simulink model "sampleModel2432"  (R2017a)
settings: Solver=VariableStepAuto  StartTime=0.0  StopTime=10.0  RelTol=1e-3
undefined symbols (not defined in the file or in its folder): DiscIntNeverNeededParam, sigbuilder_block
libraries: simulink x354
(part 3 of 6)

== system sampleModel2432/cfblk229 ==
  cfblk1 : Inport
  cfblk12 : Inport  Port=2
  cfblk13 : Inport  Port=3
  Action Port : ActionPort  ActionType=then
  cfblk10 : UnitDelay  SampleTime=-1
  cfblk11 : simulink/Discrete/Difference  ICPrevInput=0.0  OutMin=[]  OutMax=[]  OutDataTypeStr=Inherit: Inherit via back propagation  OutDataType=fixdt(1, 16)  OutScaling=2^-10  DoSatur=off
  cfblk15 : Delay
  cfblk3 : DiscreteTransferFcn
  cfblk4 : simulink/Discrete/Transfer Fcn Lead or Lag  PoleZ=0.95  ZeroZ=0.75  ICPrevOutput=0.0  ICPrevInput=0.0  DoSatur=off
      settings: SourceProductName=Simulink  SourceProductBaseCode=SL
  cfblk5 : simulink/Discrete/Tapped Delay  vinit=0.0  samptime=-1  NumDelays=1  DelayOrder=Oldest  includeCurrent=off
  cfblk6 : simulink/Continuous/PID Controller (2DOF)  Controller=PID  TimeDomain=Discrete-time  SampleTime=-1  IntegratorMethod=Forward Euler  FilterMethod=Forward Euler  Form=Parallel  UseFilter=on  ControllerParametersSource=internal  P=1  I=1  D=0  N=100  b=1  c=1  InitialConditionSource=internal  InitialConditionForIntegrator=0  InitialConditionForFilter=0  ExternalReset=none  LimitOutput=off  UpperSaturationLimit=inf  LowerSaturationLimit=-inf  LinearizeAsGain=off  AntiWindupMode=none  Kb=1  TrackingMode=off  Kt=1  PParamMin=[]  PParamMax=[]  IParamMin=[]  IParamMax=[]  DParamMin=[]  DParamMax=[]  NParamMin=[]  NParamMax=[]  bParamMin=[]  bParamMax=[]  cParamMin=[]  cParamMax=[]  KbParamMin=[]  KbParamMax=[]  KtParamMin=[]  KtParamMax=[]  POutMin=[]  POutMax=[]  IOutMin=[]  IOutMax=[]  DOutMin=[]  DOutMax=[]  NOutMin=[]  NOutMax=[]  bOutMin=[]  bOutMax=[]  cOutMin=[]  cOutMax=[]  KbOutMin=[]  KbOutMax=[]  KtOutMin=[]  KtOutMax=[]  IntegratorOutMin=[]  IntegratorOutMax=[]  FilterOutMin=[]  FilterOutMax=[]  SumOutMin=[]  SumOutMax=[]  Sum1OutMin=[]  Sum1OutMax=[]  Sum2OutMin=[]  Sum2OutMax=[]  Sum3OutMin=[]  Sum3OutMax=[]  SumI1OutMin=[]  SumI1OutMax=[]  SumI2OutMin=[]  SumI2OutMax=[]  SumI3OutMin=[]  SumI3OutMax=[]  SumDOutMin=[]  SumDOutMax=[]  SaturationOutMin=[]  SaturationOutMax=[]  IntegratorContinuousStateAttributes=''  IntegratorStateMustResolveToSignalObject=off  IntegratorRTWStateStorageClass=Auto  FilterContinuousStateAttributes=''  FilterStateMustResolveToSignalObject=off  FilterRTWStateStorageClass=Auto  DifferentiatorICPrevScaledInput=0  DifferentiatorOutMin=[]  DifferentiatorOutMax=[]  InitialConditionSetting=State (most efficient)
  cfblk7 : simulink/Continuous/PID Controller  Controller=PID  TimeDomain=Discrete-time  SampleTime=-1  IntegratorMethod=Forward Euler  FilterMethod=Forward Euler  Form=Parallel  UseFilter=on  ControllerParametersSource=internal  P=1  I=1  D=0  N=100  InitialConditionSource=internal  InitialConditionForIntegrator=0  InitialConditionForFilter=0  ExternalReset=none  LimitOutput=off  UpperSaturationLimit=inf  LowerSaturationLimit=-inf  LinearizeAsGain=off  AntiWindupMode=none  Kb=1  TrackingMode=off  Kt=1  PParamMin=[]  PParamMax=[]  IParamMin=[]  IParamMax=[]  DParamMin=[]  DParamMax=[]  NParamMin=[]  NParamMax=[]  KbParamMin=[]  KbParamMax=[]  KtParamMin=[]  KtParamMax=[]  POutMin=[]  POutMax=[]  IOutMin=[]  IOutMax=[]  DOutMin=[]  DOutMax=[]  NOutMin=[]  NOutMax=[]  KbOutMin=[]  KbOutMax=[]  KtOutMin=[]  KtOutMax=[]  IntegratorOutMin=[]  IntegratorOutMax=[]  FilterOutMin=[]  FilterOutMax=[]  SumOutMin=[]  SumOutMax=[]  SumI1OutMin=[]  SumI1OutMax=[]  SumI2OutMin=[]  SumI2OutMax=[]  SumI3OutMin=[]  SumI3OutMax=[]  SumDOutMin=[]  SumDOutMax=[]  SaturationOutMin=[]  SaturationOutMax=[]  IntegratorContinuousStateAttributes=''  IntegratorStateMustResolveToSignalObject=off  IntegratorRTWStateStorageClass=Auto  FilterContinuousStateAttributes=''  FilterStateMustResolveToSignalObject=off  FilterRTWStateStorageClass=Auto  DifferentiatorICPrevScaledInput=0  DifferentiatorOutMin=[]  DifferentiatorOutMax=[]  InitialConditionSetting=State (most efficient)
  cfblk8 : simulink/Continuous/PID Controller  Controller=PID  TimeDomain=Discrete-time  SampleTime=-1  IntegratorMethod=Forward Euler  FilterMethod=Forward Euler  Form=Parallel  UseFilter=on  ControllerParametersSource=internal  P=1  I=1  D=0  N=100  InitialConditionSource=internal  InitialConditionForIntegrator=0  InitialConditionForFilter=0  ExternalReset=none  LimitOutput=off  UpperSaturationLimit=inf  LowerSaturationLimit=-inf  LinearizeAsGain=off  AntiWindupMode=none  Kb=1  TrackingMode=off  Kt=1  PParamMin=[]  PParamMax=[]  IParamMin=[]  IParamMax=[]  DParamMin=[]  DParamMax=[]  NParamMin=[]  NParamMax=[]  KbParamMin=[]  KbParamMax=[]  KtParamMin=[]  KtParamMax=[]  POutMin=[]  POutMax=[]  IOutMin=[]  IOutMax=[]  DOutMin=[]  DOutMax=[]  NOutMin=[]  NOutMax=[]  KbOutMin=[]  KbOutMax=[]  KtOutMin=[]  KtOutMax=[]  IntegratorOutMin=[]  IntegratorOutMax=[]  FilterOutMin=[]  FilterOutMax=[]  SumOutMin=[]  SumOutMax=[]  SumI1OutMin=[]  SumI1OutMax=[]  SumI2OutMin=[]  SumI2OutMax=[]  SumI3OutMin=[]  SumI3OutMax=[]  SumDOutMin=[]  SumDOutMax=[]  SaturationOutMin=[]  SaturationOutMax=[]  IntegratorContinuousStateAttributes=''  IntegratorStateMustResolveToSignalObject=off  IntegratorRTWStateStorageClass=Auto  FilterContinuousStateAttributes=''  FilterStateMustResolveToSignalObject=off  FilterRTWStateStorageClass=Auto  DifferentiatorICPrevScaledInput=0  DifferentiatorOutMin=[]  DifferentiatorOutMax=[]  InitialConditionSetting=State (most efficient)
  cfblk9 : DiscreteZeroPole  Poles=[0 0.5]  Gain=1  SampleTime=-1
  cfblk2 : Outport
  cfblk14 : Outport  Port=2
  wires:
  cfblk7/1 -> cfblk8/1
  cfblk5/1 -> cfblk10/1
  cfblk11/1 -> cfblk7/1
  cfblk4/1 -> cfblk9/1
  cfblk8/1 -> cfblk14/1
  cfblk13/1 -> cfblk6/1
  cfblk9/1 -> cfblk5/1
  cfblk1/1 -> cfblk6/2
  cfblk6/1 -> cfblk2/1
  cfblk12/1 -> cfblk3/1
  cfblk3/1 -> cfblk11/1
  cfblk10/1 -> cfblk15/1
  cfblk15/1 -> cfblk4/1

== system sampleModel2432/cfblk230 ==
  cfblk1 : Inport
  Action Port : ActionPort  ActionType=else
  cfblk10 : Subsystem  TreatAsAtomicUnit=on
  cfblk11 : Subsystem  TreatAsAtomicUnit=on
  cfblk12 : Delay
  cfblk3 : DiscreteZeroPole  Poles=[0 0.5]  Gain=1  SampleTime=-1
  cfblk4 : Delay  DelayLengthSource=Input port
      settings: InputPortMap=u0,p1
  cfblk5 : DiscreteZeroPole  Poles=[0 0.5]  Gain=1  SampleTime=-1
  cfblk6 : simulink/Discrete/Transfer Fcn Lead or Lag  PoleZ=0.95  ZeroZ=0.75  ICPrevOutput=0.0  ICPrevInput=0.0  DoSatur=off
      settings: SourceProductName=Simulink  SourceProductBaseCode=SL
  cfblk7 : DiscreteIntegrator  InitialConditionSetting=State (most efficient)  SampleTime=-1  ICPrevOutput=DiscIntNeverNeededParam  ICPrevScaledInput=DiscIntNeverNeededParam
  cfblk8 : simulink/Continuous/PID Controller  Controller=PID  TimeDomain=Discrete-time  SampleTime=-1  IntegratorMethod=Forward Euler  FilterMethod=Forward Euler  Form=Parallel  UseFilter=on  ControllerParametersSource=internal  P=1  I=1  D=0  N=100  InitialConditionSource=internal  InitialConditionForIntegrator=0  InitialConditionForFilter=0  ExternalReset=none  LimitOutput=off  UpperSaturationLimit=inf  LowerSaturationLimit=-inf  LinearizeAsGain=off  AntiWindupMode=none  Kb=1  TrackingMode=off  Kt=1  PParamMin=[]  PParamMax=[]  IParamMin=[]  IParamMax=[]  DParamMin=[]  DParamMax=[]  NParamMin=[]  NParamMax=[]  KbParamMin=[]  KbParamMax=[]  KtParamMin=[]  KtParamMax=[]  POutMin=[]  POutMax=[]  IOutMin=[]  IOutMax=[]  DOutMin=[]  DOutMax=[]  NOutMin=[]  NOutMax=[]  KbOutMin=[]  KbOutMax=[]  KtOutMin=[]  KtOutMax=[]  IntegratorOutMin=[]  IntegratorOutMax=[]  FilterOutMin=[]  FilterOutMax=[]  SumOutMin=[]  SumOutMax=[]  SumI1OutMin=[]  SumI1OutMax=[]  SumI2OutMin=[]  SumI2OutMax=[]  SumI3OutMin=[]  SumI3OutMax=[]  SumDOutMin=[]  SumDOutMax=[]  SaturationOutMin=[]  SaturationOutMax=[]  IntegratorContinuousStateAttributes=''  IntegratorStateMustResolveToSignalObject=off  IntegratorRTWStateStorageClass=Auto  FilterContinuousStateAttributes=''  FilterStateMustResolveToSignalObject=off  FilterRTWStateStorageClass=Auto  DifferentiatorICPrevScaledInput=0  DifferentiatorOutMin=[]  DifferentiatorOutMax=[]  InitialConditionSetting=State (most efficient)
  cfblk9 : If  SampleTime=1
  cfblk2 : Outport
  wires:
  cfblk7/1 -> cfblk3/1
  cfblk10/1(cfblk2) -> cfblk7/1
  cfblk10/2(cfblk11) -> cfblk11/1(cfblk1)
  cfblk8/1 -> cfblk6/1
  cfblk5/1 -> cfblk2/1
  cfblk1/1 -> cfblk9/1
  cfblk3/1 -> cfblk5/1
  cfblk10/3(cfblk12) -> cfblk4/1
  cfblk11/1(cfblk2) -> cfblk8/1
  cfblk11/2(cfblk10) -> cfblk4/2
  cfblk9/1 -> cfblk10/Action
  cfblk9/2 -> cfblk11/Action
  cfblk6/1 -> cfblk12/1
  cfblk12/1 -> cfblk10/1(cfblk1)

== system sampleModel2432/cfblk231 ==
  cfblk1 : Inport
  cfblk11 : Inport  Port=2
  cfblk12 : Inport  Port=3
  Action Port : ActionPort  ActionType=then
  cfblk10 : If  SampleTime=1
  cfblk14 : Subsystem  TreatAsAtomicUnit=on
  cfblk15 : Subsystem  TreatAsAtomicUnit=on
  cfblk16 : Delay
  cfblk17 : Delay
  cfblk3 : Delay
  cfblk4 : simulink/Discrete/Transfer Fcn First Order  PoleZ=0.95  ICPrevOutput=0.0  DoSatur=off
      settings: SourceProductName=Simulink
  cfblk5 : simulink/Discrete/Difference  ICPrevInput=0.0  OutMin=[]  OutMax=[]  OutDataTypeStr=Inherit: Inherit via back propagation  OutDataType=fixdt(1, 16)  OutScaling=2^-10  DoSatur=off
  cfblk6 : DiscreteIntegrator  InitialConditionSetting=State (most efficient)  SampleTime=-1  ICPrevOutput=DiscIntNeverNeededParam  ICPrevScaledInput=DiscIntNeverNeededParam
  cfblk7 : DiscreteFilter
  cfblk8 : DiscreteFir
  cfblk9 : simulink/Discrete/Tapped Delay  vinit=0.0  samptime=-1  NumDelays=1  DelayOrder=Oldest  includeCurrent=off
  cfblk2 : Outport
  cfblk13 : Outport  Port=2
  wires:
  cfblk11/1 -> cfblk6/1
  cfblk5/1 -> cfblk3/1
  cfblk4/1 -> cfblk5/1
  cfblk14/1(cfblk2) -> cfblk4/1
  cfblk9/1 -> cfblk13/1
  cfblk6/1 -> cfblk14/2(cfblk6)
  cfblk1/1 -> cfblk15/1(cfblk1)
  cfblk12/1 -> cfblk14/3(cfblk7)
  cfblk15/1(cfblk2) -> cfblk8/1
  cfblk14/2(cfblk10) -> cfblk9/1
  cfblk15/2(cfblk6) -> cfblk7/1
  cfblk14/3(cfblk11) -> cfblk2/1
  cfblk15/3(cfblk7) -> cfblk14/4(cfblk8)
  cfblk15/4(cfblk8) -> cfblk14/5(cfblk9)
  cfblk10/1 -> cfblk14/Action
  cfblk10/2 -> cfblk15/Action
  cfblk3/1 -> cfblk16/1
  cfblk16/1 -> cfblk14/1(cfblk1)
  cfblk8/1 -> cfblk17/1
  cfblk17/1 -> cfblk10/1

== system sampleModel2432/cfblk232 ==
  cfblk1 : Inport
  cfblk7 : Inport  Port=2
  Action Port : ActionPort  ActionType=else
  cfblk3 : simulink/Continuous/PID Controller (2DOF)  Controller=PID  TimeDomain=Discrete-time  SampleTime=-1  IntegratorMethod=Forward Euler  FilterMethod=Forward Euler  Form=Parallel  UseFilter=on  ControllerParametersSource=internal  P=1  I=1  D=0  N=100  b=1  c=1  InitialConditionSource=internal  InitialConditionForIntegrator=0  InitialConditionForFilter=0  ExternalReset=none  LimitOutput=off  UpperSaturationLimit=inf  LowerSaturationLimit=-inf  LinearizeAsGain=off  AntiWindupMode=none  Kb=1  TrackingMode=off  Kt=1  PParamMin=[]  PParamMax=[]  IParamMin=[]  IParamMax=[]  DParamMin=[]  DParamMax=[]  NParamMin=[]  NParamMax=[]  bParamMin=[]  bParamMax=[]  cParamMin=[]  cParamMax=[]  KbParamMin=[]  KbParamMax=[]  KtParamMin=[]  KtParamMax=[]  POutMin=[]  POutMax=[]  IOutMin=[]  IOutMax=[]  DOutMin=[]  DOutMax=[]  NOutMin=[]  NOutMax=[]  bOutMin=[]  bOutMax=[]  cOutMin=[]  cOutMax=[]  KbOutMin=[]  KbOutMax=[]  KtOutMin=[]  KtOutMax=[]  IntegratorOutMin=[]  IntegratorOutMax=[]  FilterOutMin=[]  FilterOutMax=[]  SumOutMin=[]  SumOutMax=[]  Sum1OutMin=[]  Sum1OutMax=[]  Sum2OutMin=[]  Sum2OutMax=[]  Sum3OutMin=[]  Sum3OutMax=[]  SumI1OutMin=[]  SumI1OutMax=[]  SumI2OutMin=[]  SumI2OutMax=[]  SumI3OutMin=[]  SumI3OutMax=[]  SumDOutMin=[]  SumDOutMax=[]  SaturationOutMin=[]  SaturationOutMax=[]  IntegratorContinuousStateAttributes=''  IntegratorStateMustResolveToSignalObject=off  IntegratorRTWStateStorageClass=Auto  FilterContinuousStateAttributes=''  FilterStateMustResolveToSignalObject=off  FilterRTWStateStorageClass=Auto  DifferentiatorICPrevScaledInput=0  DifferentiatorOutMin=[]  DifferentiatorOutMax=[]  InitialConditionSetting=State (most efficient)
  cfblk4 : simulink/Discrete/Transfer Fcn First Order  PoleZ=0.95  ICPrevOutput=0.0  DoSatur=off
      settings: SourceProductName=Simulink
  cfblk5 : Delay
  cfblk6 : simulink/Discrete/Difference  ICPrevInput=0.0  OutMin=[]  OutMax=[]  OutDataTypeStr=Inherit: Inherit via back propagation  OutDataType=fixdt(1, 16)  OutScaling=2^-10  DoSatur=off
  cfblk8 : Delay
  cfblk2 : Outport
  wires:
  cfblk4/1 -> cfblk6/1
  cfblk7/1 -> cfblk3/1
  cfblk3/1 -> cfblk2/1
  cfblk1/1 -> cfblk5/1
  cfblk5/1 -> cfblk3/2
  cfblk6/1 -> cfblk8/1
  cfblk8/1 -> cfblk4/1

== system sampleModel2432/cfblk233 ==
  cfblk1 : Inport
  Action Port : ActionPort  ActionType=then
  cfblk10 : DiscreteIntegrator  InitialConditionSetting=State (most efficient)  SampleTime=-1  ICPrevOutput=DiscIntNeverNeededParam  ICPrevScaledInput=DiscIntNeverNeededParam
  cfblk{5,8..9,11..12} (5 alike) : DiscreteFir
  cfblk13 : simulink/Continuous/PID Controller  Controller=PID  TimeDomain=Discrete-time  SampleTime=-1  IntegratorMethod=Forward Euler  FilterMethod=Forward Euler  Form=Parallel  UseFilter=on  ControllerParametersSource=internal  P=1  I=1  D=0  N=100  InitialConditionSource=internal  InitialConditionForIntegrator=0  InitialConditionForFilter=0  ExternalReset=none  LimitOutput=off  UpperSaturationLimit=inf  LowerSaturationLimit=-inf  LinearizeAsGain=off  AntiWindupMode=none  Kb=1  TrackingMode=off  Kt=1  PParamMin=[]  PParamMax=[]  IParamMin=[]  IParamMax=[]  DParamMin=[]  DParamMax=[]  NParamMin=[]  NParamMax=[]  KbParamMin=[]  KbParamMax=[]  KtParamMin=[]  KtParamMax=[]  POutMin=[]  POutMax=[]  IOutMin=[]  IOutMax=[]  DOutMin=[]  DOutMax=[]  NOutMin=[]  NOutMax=[]  KbOutMin=[]  KbOutMax=[]  KtOutMin=[]  KtOutMax=[]  IntegratorOutMin=[]  IntegratorOutMax=[]  FilterOutMin=[]  FilterOutMax=[]  SumOutMin=[]  SumOutMax=[]  SumI1OutMin=[]  SumI1OutMax=[]  SumI2OutMin=[]  SumI2OutMax=[]  SumI3OutMin=[]  SumI3OutMax=[]  SumDOutMin=[]  SumDOutMax=[]  SaturationOutMin=[]  SaturationOutMax=[]  IntegratorContinuousStateAttributes=''  IntegratorStateMustResolveToSignalObject=off  IntegratorRTWStateStorageClass=Auto  FilterContinuousStateAttributes=''  FilterStateMustResolveToSignalObject=off  FilterRTWStateStorageClass=Auto  DifferentiatorICPrevScaledInput=0  DifferentiatorOutMin=[]  DifferentiatorOutMax=[]  InitialConditionSetting=State (most efficient)
  cfblk14 : DiscreteZeroPole  Poles=[0 0.5]  Gain=1  SampleTime=-1
  cfblk15 : Delay
  cfblk16 : Delay
  cfblk3 : simulink/Discrete/Tapped Delay  vinit=0.0  samptime=-1  NumDelays=1  DelayOrder=Oldest  includeCurrent=off
  cfblk4 : simulink/Discrete/Transfer Fcn First Order  PoleZ=0.95  ICPrevOutput=0.0  DoSatur=off
      settings: SourceProductName=Simulink
  cfblk6 : simulink/Discrete/Transfer Fcn Lead or Lag  PoleZ=0.95  ZeroZ=0.75  ICPrevOutput=0.0  ICPrevInput=0.0  DoSatur=off
      settings: SourceProductName=Simulink  SourceProductBaseCode=SL
  cfblk7 : simulink/Discrete/Transfer Fcn Lead or Lag  PoleZ=0.95  ZeroZ=0.75  ICPrevOutput=0.0  ICPrevInput=0.0  DoSatur=off
      settings: SourceProductName=Simulink  SourceProductBaseCode=SL
  cfblk2 : Outport
  wires:
  cfblk14/1 -> cfblk9/1
  cfblk3/1 -> cfblk12/1
  cfblk7/1 -> cfblk6/1
  cfblk9/1 -> cfblk10/1
  cfblk12/1 -> cfblk2/1
  cfblk8/1 -> cfblk11/1
  cfblk6/1 -> cfblk13/1
  cfblk4/1 -> cfblk14/1
  cfblk5/1 -> cfblk8/1
  cfblk1/1 -> cfblk3/1
  cfblk10/1 -> cfblk7/1
  cfblk13/1 -> cfblk15/1
  cfblk15/1 -> cfblk4/1
  cfblk11/1 -> cfblk16/1
  cfblk16/1 -> cfblk5/1

== system sampleModel2432/cfblk234 ==
  cfblk1 : Inport
  cfblk7 : Inport  Port=2
  Action Port : ActionPort  ActionType=else
  cfblk10 : Delay
  cfblk11 : Delay
  cfblk3 : simulink/Discrete/Difference  ICPrevInput=0.0  OutMin=[]  OutMax=[]  OutDataTypeStr=Inherit: Inherit via back propagation  OutDataType=fixdt(1, 16)  OutScaling=2^-10  DoSatur=off
  cfblk4 : simulink/Discrete/Difference  ICPrevInput=0.0  OutMin=[]  OutMax=[]  OutDataTypeStr=Inherit: Inherit via back propagation  OutDataType=fixdt(1, 16)  OutScaling=2^-10  DoSatur=off
  cfblk5 : Delay
  cfblk6 : If  SampleTime=1
  cfblk8 : Subsystem  TreatAsAtomicUnit=on
  cfblk9 : Subsystem  TreatAsAtomicUnit=on
  cfblk2 : Outport
  wires:
  cfblk8/1(cfblk2) -> cfblk5/1
  cfblk7/1 -> cfblk8/1(cfblk1)
  cfblk4/1 -> cfblk2/1
  cfblk1/1 -> cfblk4/1
  cfblk3/1 -> cfblk9/1(cfblk1)
  cfblk6/1 -> cfblk8/Action
  cfblk6/2 -> cfblk9/Action
  cfblk5/1 -> cfblk10/1
  cfblk10/1 -> cfblk3/1
  cfblk9/1(cfblk2) -> cfblk11/1
  cfblk11/1 -> cfblk6/1

== system sampleModel2432/cfblk235 ==
  cfblk1 : Inport
  Action Port : ActionPort  ActionType=then
  cfblk10 : Delay
  cfblk3 : Delay  ShowEnablePort=on
      settings: InputPortMap=u0,e6
  cfblk4 : DiscreteIntegrator  InitialConditionSetting=State (most efficient)  SampleTime=-1  ICPrevOutput=DiscIntNeverNeededParam  ICPrevScaledInput=DiscIntNeverNeededParam
  cfblk5 : simulink/Continuous/PID Controller  Controller=PID  TimeDomain=Discrete-time  SampleTime=-1  IntegratorMethod=Forward Euler  FilterMethod=Forward Euler  Form=Parallel  UseFilter=on  ControllerParametersSource=internal  P=1  I=1  D=0  N=100  InitialConditionSource=internal  InitialConditionForIntegrator=0  InitialConditionForFilter=0  ExternalReset=none  LimitOutput=off  UpperSaturationLimit=inf  LowerSaturationLimit=-inf  LinearizeAsGain=off  AntiWindupMode=none  Kb=1  TrackingMode=off  Kt=1  PParamMin=[]  PParamMax=[]  IParamMin=[]  IParamMax=[]  DParamMin=[]  DParamMax=[]  NParamMin=[]  NParamMax=[]  KbParamMin=[]  KbParamMax=[]  KtParamMin=[]  KtParamMax=[]  POutMin=[]  POutMax=[]  IOutMin=[]  IOutMax=[]  DOutMin=[]  DOutMax=[]  NOutMin=[]  NOutMax=[]  KbOutMin=[]  KbOutMax=[]  KtOutMin=[]  KtOutMax=[]  IntegratorOutMin=[]  IntegratorOutMax=[]  FilterOutMin=[]  FilterOutMax=[]  SumOutMin=[]  SumOutMax=[]  SumI1OutMin=[]  SumI1OutMax=[]  SumI2OutMin=[]  SumI2OutMax=[]  SumI3OutMin=[]  SumI3OutMax=[]  SumDOutMin=[]  SumDOutMax=[]  SaturationOutMin=[]  SaturationOutMax=[]  IntegratorContinuousStateAttributes=''  IntegratorStateMustResolveToSignalObject=off  IntegratorRTWStateStorageClass=Auto  FilterContinuousStateAttributes=''  FilterStateMustResolveToSignalObject=off  FilterRTWStateStorageClass=Auto  DifferentiatorICPrevScaledInput=0  DifferentiatorOutMin=[]  DifferentiatorOutMax=[]  InitialConditionSetting=State (most efficient)
  cfblk6 : Delay  ShowEnablePort=on
      settings: InputPortMap=u0,e6
  cfblk7 : Delay
  cfblk9 : Delay
  cfblk2 : Outport
  cfblk8 : Outport  Port=2
  wires:
  cfblk1/1 -> cfblk6/1, cfblk2/1
  cfblk7/1 -> cfblk8/1, cfblk6/2, cfblk10/1
  cfblk3/1 -> cfblk5/1
  cfblk4/1 -> cfblk7/1
  cfblk6/1 -> cfblk3/2
  cfblk5/1 -> cfblk9/1
  cfblk9/1 -> cfblk3/1
  cfblk10/1 -> cfblk4/1

== system sampleModel2432/cfblk236 ==
  cfblk1 : Inport
  Action Port : ActionPort  ActionType=else
  cfblk{9..12} (4 alike) : DiscreteIntegrator  InitialConditionSetting=State (most efficient)  SampleTime=-1  ICPrevOutput=DiscIntNeverNeededParam  ICPrevScaledInput=DiscIntNeverNeededParam
  cfblk13 : simulink/Discrete/Transfer Fcn First Order  PoleZ=0.95  ICPrevOutput=0.0  DoSatur=off
      settings: SourceProductName=Simulink
  cfblk3 : simulink/Continuous/PID Controller  Controller=PID  TimeDomain=Discrete-time  SampleTime=-1  IntegratorMethod=Forward Euler  FilterMethod=Forward Euler  Form=Parallel  UseFilter=on  ControllerParametersSource=internal  P=1  I=1  D=0  N=100  InitialConditionSource=internal  InitialConditionForIntegrator=0  InitialConditionForFilter=0  ExternalReset=none  LimitOutput=off  UpperSaturationLimit=inf  LowerSaturationLimit=-inf  LinearizeAsGain=off  AntiWindupMode=none  Kb=1  TrackingMode=off  Kt=1  PParamMin=[]  PParamMax=[]  IParamMin=[]  IParamMax=[]  DParamMin=[]  DParamMax=[]  NParamMin=[]  NParamMax=[]  KbParamMin=[]  KbParamMax=[]  KtParamMin=[]  KtParamMax=[]  POutMin=[]  POutMax=[]  IOutMin=[]  IOutMax=[]  DOutMin=[]  DOutMax=[]  NOutMin=[]  NOutMax=[]  KbOutMin=[]  KbOutMax=[]  KtOutMin=[]  KtOutMax=[]  IntegratorOutMin=[]  IntegratorOutMax=[]  FilterOutMin=[]  FilterOutMax=[]  SumOutMin=[]  SumOutMax=[]  SumI1OutMin=[]  SumI1OutMax=[]  SumI2OutMin=[]  SumI2OutMax=[]  SumI3OutMin=[]  SumI3OutMax=[]  SumDOutMin=[]  SumDOutMax=[]  SaturationOutMin=[]  SaturationOutMax=[]  IntegratorContinuousStateAttributes=''  IntegratorStateMustResolveToSignalObject=off  IntegratorRTWStateStorageClass=Auto  FilterContinuousStateAttributes=''  FilterStateMustResolveToSignalObject=off  FilterRTWStateStorageClass=Auto  DifferentiatorICPrevScaledInput=0  DifferentiatorOutMin=[]  DifferentiatorOutMax=[]  InitialConditionSetting=State (most efficient)
  cfblk4 : simulink/Discrete/Tapped Delay  vinit=0.0  samptime=-1  NumDelays=1  DelayOrder=Oldest  includeCurrent=off
  cfblk5 : Delay  DelayLengthSource=Input port
      settings: InputPortMap=u0,p1
  cfblk6 : Delay  ShowEnablePort=on
      settings: InputPortMap=u0,e6
  cfblk7 : Delay
  cfblk8 : DiscreteTransferFcn
  cfblk2 : Outport
  wires:
  cfblk3/1 -> cfblk4/1, cfblk13/1
  cfblk1/1 -> cfblk3/1, cfblk6/2
  cfblk9/1 -> cfblk8/1
  cfblk8/1 -> cfblk10/1
  cfblk5/1 -> cfblk2/1
  cfblk12/1 -> cfblk11/1
  cfblk10/1 -> cfblk12/1
  cfblk7/1 -> cfblk5/1
  cfblk6/1 -> cfblk7/1
  cfblk13/1 -> cfblk9/1
  cfblk4/1 -> cfblk6/1
  cfblk11/1 -> cfblk5/2

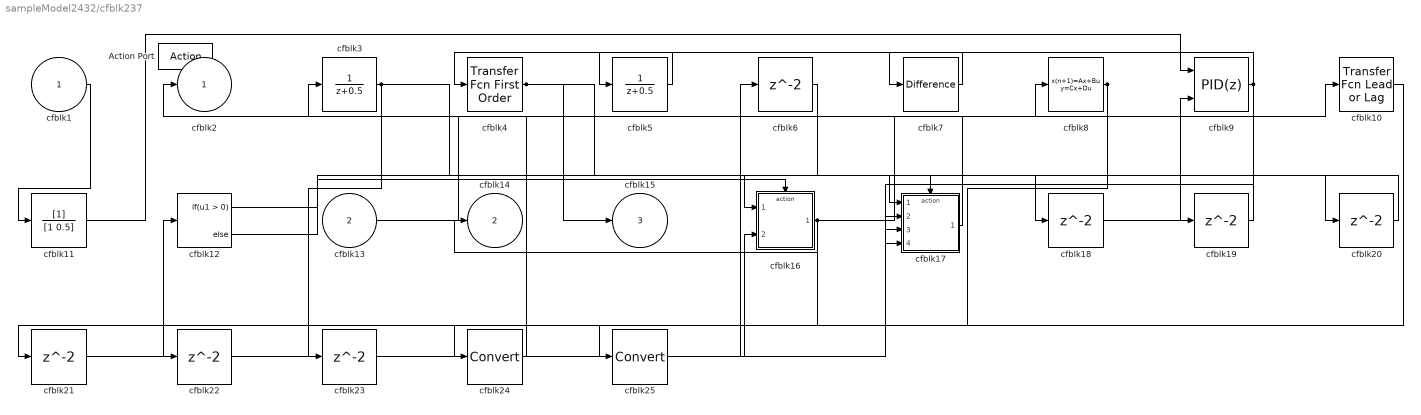
== system sampleModel2432/cfblk237 ==
  cfblk1 : Inport
  cfblk13 : Inport  Port=2
  Action Port : ActionPort  ActionType=then
  cfblk10 : simulink/Discrete/Transfer Fcn Lead or Lag  PoleZ=0.95  ZeroZ=0.75  ICPrevOutput=0.0  ICPrevInput=0.0  DoSatur=off
      settings: SourceProductName=Simulink  SourceProductBaseCode=SL
  cfblk11 : DiscreteFilter
  cfblk12 : If  SampleTime=1
  cfblk16 : Subsystem  TreatAsAtomicUnit=on
  cfblk17 : Subsystem  TreatAsAtomicUnit=on
  cfblk{6,18..23} (7 alike) : Delay
  cfblk24 : DataTypeConversion
  cfblk25 : DataTypeConversion
  cfblk3 : DiscreteTransferFcn
  cfblk4 : simulink/Discrete/Transfer Fcn First Order  PoleZ=0.95  ICPrevOutput=0.0  DoSatur=off
      settings: SourceProductName=Simulink
  cfblk5 : DiscreteTransferFcn
  cfblk7 : simulink/Discrete/Difference  ICPrevInput=0.0  OutMin=[]  OutMax=[]  OutDataTypeStr=Inherit: Inherit via back propagation  OutDataType=fixdt(1, 16)  OutScaling=2^-10  DoSatur=off
  cfblk8 : DiscreteStateSpace  SampleTime=-1
  cfblk9 : simulink/Continuous/PID Controller (2DOF)  Controller=PID  TimeDomain=Discrete-time  SampleTime=-1  IntegratorMethod=Forward Euler  FilterMethod=Forward Euler  Form=Parallel  UseFilter=on  ControllerParametersSource=internal  P=1  I=1  D=0  N=100  b=1  c=1  InitialConditionSource=internal  InitialConditionForIntegrator=0  InitialConditionForFilter=0  ExternalReset=none  LimitOutput=off  UpperSaturationLimit=inf  LowerSaturationLimit=-inf  LinearizeAsGain=off  AntiWindupMode=none  Kb=1  TrackingMode=off  Kt=1  PParamMin=[]  PParamMax=[]  IParamMin=[]  IParamMax=[]  DParamMin=[]  DParamMax=[]  NParamMin=[]  NParamMax=[]  bParamMin=[]  bParamMax=[]  cParamMin=[]  cParamMax=[]  KbParamMin=[]  KbParamMax=[]  KtParamMin=[]  KtParamMax=[]  POutMin=[]  POutMax=[]  IOutMin=[]  IOutMax=[]  DOutMin=[]  DOutMax=[]  NOutMin=[]  NOutMax=[]  bOutMin=[]  bOutMax=[]  cOutMin=[]  cOutMax=[]  KbOutMin=[]  KbOutMax=[]  KtOutMin=[]  KtOutMax=[]  IntegratorOutMin=[]  IntegratorOutMax=[]  FilterOutMin=[]  FilterOutMax=[]  SumOutMin=[]  SumOutMax=[]  Sum1OutMin=[]  Sum1OutMax=[]  Sum2OutMin=[]  Sum2OutMax=[]  Sum3OutMin=[]  Sum3OutMax=[]  SumI1OutMin=[]  SumI1OutMax=[]  SumI2OutMin=[]  SumI2OutMax=[]  SumI3OutMin=[]  SumI3OutMax=[]  SumDOutMin=[]  SumDOutMax=[]  SaturationOutMin=[]  SaturationOutMax=[]  IntegratorContinuousStateAttributes=''  IntegratorStateMustResolveToSignalObject=off  IntegratorRTWStateStorageClass=Auto  FilterContinuousStateAttributes=''  FilterStateMustResolveToSignalObject=off  FilterRTWStateStorageClass=Auto  DifferentiatorICPrevScaledInput=0  DifferentiatorOutMin=[]  DifferentiatorOutMax=[]  InitialConditionSetting=State (most efficient)
  cfblk2 : Outport
  cfblk14 : Outport  Port=2
  cfblk15 : Outport  Port=3
  wires:
  cfblk4/1 -> cfblk15/1, cfblk18/1
  cfblk1/1 -> cfblk11/1
  cfblk5/1 -> cfblk4/1
  cfblk16/1(cfblk2) -> cfblk10/1, cfblk14/1, cfblk22/1
  cfblk8/1 -> cfblk17/2(cfblk10), cfblk25/1
  cfblk7/1 -> cfblk5/1
  cfblk13/1 -> cfblk8/1
  cfblk11/1 -> cfblk9/1
  cfblk17/1(cfblk2) -> cfblk3/1
  cfblk9/1 -> cfblk7/1, cfblk17/4(cfblk12)
  cfblk3/1 -> cfblk19/1, cfblk20/1, cfblk23/1
  cfblk12/1 -> cfblk16/Action
  cfblk12/2 -> cfblk17/Action
  cfblk18/1 -> cfblk9/2
  cfblk19/1 -> cfblk17/1(cfblk1)
  cfblk20/1 -> cfblk16/1(cfblk1)
  cfblk10/1 -> cfblk21/1
  cfblk21/1 -> cfblk12/1
  cfblk22/1 -> cfblk17/3(cfblk11)
  cfblk23/1 -> cfblk16/2(cfblk16)
  cfblk6/1 -> cfblk24/1
  cfblk24/1 -> cfblk2/1
  cfblk25/1 -> cfblk6/1

== system sampleModel2432/cfblk238 ==
  cfblk1 : Inport
  cfblk12 : Inport  Port=2
  Action Port : ActionPort  ActionType=else
  cfblk10 : DiscreteIntegrator  InitialConditionSetting=State (most efficient)  SampleTime=-1  ICPrevOutput=DiscIntNeverNeededParam  ICPrevScaledInput=DiscIntNeverNeededParam
  cfblk11 : Delay  ShowEnablePort=on
      settings: InputPortMap=u0,e6
  cfblk16 : Delay
  cfblk17 : Delay
  cfblk3 : DiscreteFilter
  cfblk4 : simulink/Discrete/Difference  ICPrevInput=0.0  OutMin=[]  OutMax=[]  OutDataTypeStr=Inherit: Inherit via back propagation  OutDataType=fixdt(1, 16)  OutScaling=2^-10  DoSatur=off
  cfblk5 : simulink/Continuous/PID Controller  Controller=PID  TimeDomain=Discrete-time  SampleTime=-1  IntegratorMethod=Forward Euler  FilterMethod=Forward Euler  Form=Parallel  UseFilter=on  ControllerParametersSource=internal  P=1  I=1  D=0  N=100  InitialConditionSource=internal  InitialConditionForIntegrator=0  InitialConditionForFilter=0  ExternalReset=none  LimitOutput=off  UpperSaturationLimit=inf  LowerSaturationLimit=-inf  LinearizeAsGain=off  AntiWindupMode=none  Kb=1  TrackingMode=off  Kt=1  PParamMin=[]  PParamMax=[]  IParamMin=[]  IParamMax=[]  DParamMin=[]  DParamMax=[]  NParamMin=[]  NParamMax=[]  KbParamMin=[]  KbParamMax=[]  KtParamMin=[]  KtParamMax=[]  POutMin=[]  POutMax=[]  IOutMin=[]  IOutMax=[]  DOutMin=[]  DOutMax=[]  NOutMin=[]  NOutMax=[]  KbOutMin=[]  KbOutMax=[]  KtOutMin=[]  KtOutMax=[]  IntegratorOutMin=[]  IntegratorOutMax=[]  FilterOutMin=[]  FilterOutMax=[]  SumOutMin=[]  SumOutMax=[]  SumI1OutMin=[]  SumI1OutMax=[]  SumI2OutMin=[]  SumI2OutMax=[]  SumI3OutMin=[]  SumI3OutMax=[]  SumDOutMin=[]  SumDOutMax=[]  SaturationOutMin=[]  SaturationOutMax=[]  IntegratorContinuousStateAttributes=''  IntegratorStateMustResolveToSignalObject=off  IntegratorRTWStateStorageClass=Auto  FilterContinuousStateAttributes=''  FilterStateMustResolveToSignalObject=off  FilterRTWStateStorageClass=Auto  DifferentiatorICPrevScaledInput=0  DifferentiatorOutMin=[]  DifferentiatorOutMax=[]  InitialConditionSetting=State (most efficient)
  cfblk6 : simulink/Continuous/PID Controller (2DOF)  Controller=PID  TimeDomain=Discrete-time  SampleTime=-1  IntegratorMethod=Forward Euler  FilterMethod=Forward Euler  Form=Parallel  UseFilter=on  ControllerParametersSource=internal  P=1  I=1  D=0  N=100  b=1  c=1  InitialConditionSource=internal  InitialConditionForIntegrator=0  InitialConditionForFilter=0  ExternalReset=none  LimitOutput=off  UpperSaturationLimit=inf  LowerSaturationLimit=-inf  LinearizeAsGain=off  AntiWindupMode=none  Kb=1  TrackingMode=off  Kt=1  PParamMin=[]  PParamMax=[]  IParamMin=[]  IParamMax=[]  DParamMin=[]  DParamMax=[]  NParamMin=[]  NParamMax=[]  bParamMin=[]  bParamMax=[]  cParamMin=[]  cParamMax=[]  KbParamMin=[]  KbParamMax=[]  KtParamMin=[]  KtParamMax=[]  POutMin=[]  POutMax=[]  IOutMin=[]  IOutMax=[]  DOutMin=[]  DOutMax=[]  NOutMin=[]  NOutMax=[]  bOutMin=[]  bOutMax=[]  cOutMin=[]  cOutMax=[]  KbOutMin=[]  KbOutMax=[]  KtOutMin=[]  KtOutMax=[]  IntegratorOutMin=[]  IntegratorOutMax=[]  FilterOutMin=[]  FilterOutMax=[]  SumOutMin=[]  SumOutMax=[]  Sum1OutMin=[]  Sum1OutMax=[]  Sum2OutMin=[]  Sum2OutMax=[]  Sum3OutMin=[]  Sum3OutMax=[]  SumI1OutMin=[]  SumI1OutMax=[]  SumI2OutMin=[]  SumI2OutMax=[]  SumI3OutMin=[]  SumI3OutMax=[]  SumDOutMin=[]  SumDOutMax=[]  SaturationOutMin=[]  SaturationOutMax=[]  IntegratorContinuousStateAttributes=''  IntegratorStateMustResolveToSignalObject=off  IntegratorRTWStateStorageClass=Auto  FilterContinuousStateAttributes=''  FilterStateMustResolveToSignalObject=off  FilterRTWStateStorageClass=Auto  DifferentiatorICPrevScaledInput=0  DifferentiatorOutMin=[]  DifferentiatorOutMax=[]  InitialConditionSetting=State (most efficient)
  cfblk7 : simulink/Discrete/Transfer Fcn First Order  PoleZ=0.95  ICPrevOutput=0.0  DoSatur=off
      settings: SourceProductName=Simulink
  cfblk8 : simulink/Discrete/Transfer Fcn First Order  PoleZ=0.95  ICPrevOutput=0.0  DoSatur=off
      settings: SourceProductName=Simulink
  cfblk9 : UnitDelay  SampleTime=-1
  cfblk2 : Outport
  cfblk13 : Outport  Port=2
  cfblk14 : Outport  Port=3
  cfblk15 : Outport  Port=4
  wires:
  cfblk5/1 -> cfblk11/1
  cfblk6/1 -> cfblk15/1, cfblk16/1
  cfblk9/1 -> cfblk14/1
  cfblk11/1 -> cfblk7/1, cfblk10/1, cfblk6/2
  cfblk4/1 -> cfblk5/1
  cfblk1/1 -> cfblk8/1
  cfblk3/1 -> cfblk2/1, cfblk4/1
  cfblk12/1 -> cfblk13/1
  cfblk7/1 -> cfblk6/1
  cfblk8/1 -> cfblk9/1
  cfblk16/1 -> cfblk11/2
  cfblk10/1 -> cfblk17/1
  cfblk17/1 -> cfblk3/1

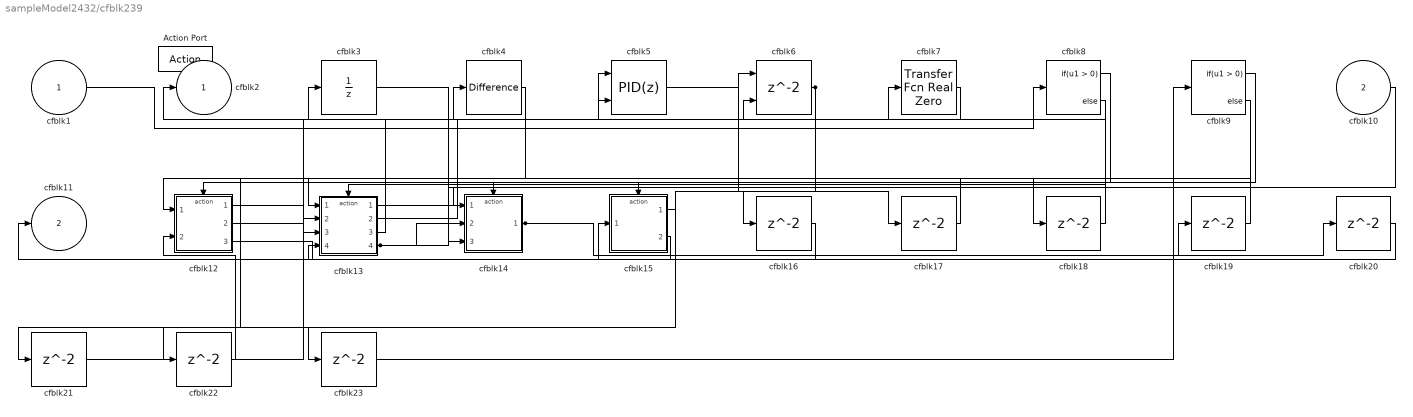
== system sampleModel2432/cfblk239 ==
  cfblk1 : Inport
  cfblk10 : Inport  Port=2
  Action Port : ActionPort  ActionType=then
  cfblk12 : Subsystem  TreatAsAtomicUnit=on
  cfblk13 : Subsystem  TreatAsAtomicUnit=on
  cfblk14 : Subsystem  TreatAsAtomicUnit=on
  cfblk15 : Subsystem  TreatAsAtomicUnit=on
  cfblk{16..23} (8 alike) : Delay
  cfblk3 : UnitDelay  SampleTime=-1
  cfblk4 : simulink/Discrete/Difference  ICPrevInput=0.0  OutMin=[]  OutMax=[]  OutDataTypeStr=Inherit: Inherit via back propagation  OutDataType=fixdt(1, 16)  OutScaling=2^-10  DoSatur=off
  cfblk5 : simulink/Continuous/PID Controller (2DOF)  Controller=PID  TimeDomain=Discrete-time  SampleTime=-1  IntegratorMethod=Forward Euler  FilterMethod=Forward Euler  Form=Parallel  UseFilter=on  ControllerParametersSource=internal  P=1  I=1  D=0  N=100  b=1  c=1  InitialConditionSource=internal  InitialConditionForIntegrator=0  InitialConditionForFilter=0  ExternalReset=none  LimitOutput=off  UpperSaturationLimit=inf  LowerSaturationLimit=-inf  LinearizeAsGain=off  AntiWindupMode=none  Kb=1  TrackingMode=off  Kt=1  PParamMin=[]  PParamMax=[]  IParamMin=[]  IParamMax=[]  DParamMin=[]  DParamMax=[]  NParamMin=[]  NParamMax=[]  bParamMin=[]  bParamMax=[]  cParamMin=[]  cParamMax=[]  KbParamMin=[]  KbParamMax=[]  KtParamMin=[]  KtParamMax=[]  POutMin=[]  POutMax=[]  IOutMin=[]  IOutMax=[]  DOutMin=[]  DOutMax=[]  NOutMin=[]  NOutMax=[]  bOutMin=[]  bOutMax=[]  cOutMin=[]  cOutMax=[]  KbOutMin=[]  KbOutMax=[]  KtOutMin=[]  KtOutMax=[]  IntegratorOutMin=[]  IntegratorOutMax=[]  FilterOutMin=[]  FilterOutMax=[]  SumOutMin=[]  SumOutMax=[]  Sum1OutMin=[]  Sum1OutMax=[]  Sum2OutMin=[]  Sum2OutMax=[]  Sum3OutMin=[]  Sum3OutMax=[]  SumI1OutMin=[]  SumI1OutMax=[]  SumI2OutMin=[]  SumI2OutMax=[]  SumI3OutMin=[]  SumI3OutMax=[]  SumDOutMin=[]  SumDOutMax=[]  SaturationOutMin=[]  SaturationOutMax=[]  IntegratorContinuousStateAttributes=''  IntegratorStateMustResolveToSignalObject=off  IntegratorRTWStateStorageClass=Auto  FilterContinuousStateAttributes=''  FilterStateMustResolveToSignalObject=off  FilterRTWStateStorageClass=Auto  DifferentiatorICPrevScaledInput=0  DifferentiatorOutMin=[]  DifferentiatorOutMax=[]  InitialConditionSetting=State (most efficient)
  cfblk6 : Delay  ShowEnablePort=on
      settings: InputPortMap=u0,e6
  cfblk7 : simulink/Discrete/Transfer Fcn Real Zero  ZeroZ=0.75  ICPrevInput=0.0  DoSatur=off
      settings: SourceProductName=Simulink  SourceProductBaseCode=SL
  cfblk8 : If  SampleTime=1
  cfblk9 : If  SampleTime=1
  cfblk2 : Outport
  cfblk11 : Outport  Port=2
  wires:
  cfblk7/1 -> cfblk2/1
  cfblk1/1 -> cfblk8/1
  cfblk14/1(cfblk2) -> cfblk19/1, cfblk20/1
  cfblk15/2(cfblk11) -> cfblk11/1
  cfblk12/1(cfblk2) -> cfblk6/2
  cfblk13/1(cfblk2) -> cfblk5/1
  cfblk6/1 -> cfblk14/3(cfblk13), cfblk16/1, cfblk21/1
  cfblk12/2(cfblk13) -> cfblk4/1
  cfblk13/2(cfblk14) -> cfblk5/2
  cfblk12/3(cfblk14) -> cfblk15/1(cfblk1)
  cfblk10/1 -> cfblk14/1(cfblk1)
  cfblk13/3(cfblk15) -> cfblk3/1
  cfblk13/4(cfblk16) -> cfblk7/1, cfblk14/2(cfblk12)
  cfblk8/1 -> cfblk12/Action
  cfblk8/2 -> cfblk13/Action
  cfblk9/1 -> cfblk14/Action
  cfblk9/2 -> cfblk15/Action
  cfblk16/1 -> cfblk13/2(cfblk11)
  cfblk5/1 -> cfblk17/1
  cfblk17/1 -> cfblk12/1(cfblk1)
  cfblk3/1 -> cfblk18/1
  cfblk18/1 -> cfblk6/1
  cfblk19/1 -> cfblk13/1(cfblk1)
  cfblk20/1 -> cfblk13/4(cfblk13)
  cfblk21/1 -> cfblk13/3(cfblk12)
  cfblk4/1 -> cfblk22/1
  cfblk22/1 -> cfblk12/2(cfblk12)
  cfblk15/1(cfblk2) -> cfblk23/1
  cfblk23/1 -> cfblk9/1

== system sampleModel2432/cfblk240 ==
  cfblk1 : Inport
  cfblk7 : Inport  Port=2
  Action Port : ActionPort  ActionType=else
  cfblk3 : simulink/Discrete/Tapped Delay  vinit=0.0  samptime=-1  NumDelays=1  DelayOrder=Oldest  includeCurrent=off
  cfblk4 : DiscreteTransferFcn
  cfblk5 : simulink/Continuous/PID Controller  Controller=PID  TimeDomain=Discrete-time  SampleTime=-1  IntegratorMethod=Forward Euler  FilterMethod=Forward Euler  Form=Parallel  UseFilter=on  ControllerParametersSource=internal  P=1  I=1  D=0  N=100  InitialConditionSource=internal  InitialConditionForIntegrator=0  InitialConditionForFilter=0  ExternalReset=none  LimitOutput=off  UpperSaturationLimit=inf  LowerSaturationLimit=-inf  LinearizeAsGain=off  AntiWindupMode=none  Kb=1  TrackingMode=off  Kt=1  PParamMin=[]  PParamMax=[]  IParamMin=[]  IParamMax=[]  DParamMin=[]  DParamMax=[]  NParamMin=[]  NParamMax=[]  KbParamMin=[]  KbParamMax=[]  KtParamMin=[]  KtParamMax=[]  POutMin=[]  POutMax=[]  IOutMin=[]  IOutMax=[]  DOutMin=[]  DOutMax=[]  NOutMin=[]  NOutMax=[]  KbOutMin=[]  KbOutMax=[]  KtOutMin=[]  KtOutMax=[]  IntegratorOutMin=[]  IntegratorOutMax=[]  FilterOutMin=[]  FilterOutMax=[]  SumOutMin=[]  SumOutMax=[]  SumI1OutMin=[]  SumI1OutMax=[]  SumI2OutMin=[]  SumI2OutMax=[]  SumI3OutMin=[]  SumI3OutMax=[]  SumDOutMin=[]  SumDOutMax=[]  SaturationOutMin=[]  SaturationOutMax=[]  IntegratorContinuousStateAttributes=''  IntegratorStateMustResolveToSignalObject=off  IntegratorRTWStateStorageClass=Auto  FilterContinuousStateAttributes=''  FilterStateMustResolveToSignalObject=off  FilterRTWStateStorageClass=Auto  DifferentiatorICPrevScaledInput=0  DifferentiatorOutMin=[]  DifferentiatorOutMax=[]  InitialConditionSetting=State (most efficient)
  cfblk6 : simulink/Continuous/PID Controller  Controller=PID  TimeDomain=Discrete-time  SampleTime=-1  IntegratorMethod=Forward Euler  FilterMethod=Forward Euler  Form=Parallel  UseFilter=on  ControllerParametersSource=internal  P=1  I=1  D=0  N=100  InitialConditionSource=internal  InitialConditionForIntegrator=0  InitialConditionForFilter=0  ExternalReset=none  LimitOutput=off  UpperSaturationLimit=inf  LowerSaturationLimit=-inf  LinearizeAsGain=off  AntiWindupMode=none  Kb=1  TrackingMode=off  Kt=1  PParamMin=[]  PParamMax=[]  IParamMin=[]  IParamMax=[]  DParamMin=[]  DParamMax=[]  NParamMin=[]  NParamMax=[]  KbParamMin=[]  KbParamMax=[]  KtParamMin=[]  KtParamMax=[]  POutMin=[]  POutMax=[]  IOutMin=[]  IOutMax=[]  DOutMin=[]  DOutMax=[]  NOutMin=[]  NOutMax=[]  KbOutMin=[]  KbOutMax=[]  KtOutMin=[]  KtOutMax=[]  IntegratorOutMin=[]  IntegratorOutMax=[]  FilterOutMin=[]  FilterOutMax=[]  SumOutMin=[]  SumOutMax=[]  SumI1OutMin=[]  SumI1OutMax=[]  SumI2OutMin=[]  SumI2OutMax=[]  SumI3OutMin=[]  SumI3OutMax=[]  SumDOutMin=[]  SumDOutMax=[]  SaturationOutMin=[]  SaturationOutMax=[]  IntegratorContinuousStateAttributes=''  IntegratorStateMustResolveToSignalObject=off  IntegratorRTWStateStorageClass=Auto  FilterContinuousStateAttributes=''  FilterStateMustResolveToSignalObject=off  FilterRTWStateStorageClass=Auto  DifferentiatorICPrevScaledInput=0  DifferentiatorOutMin=[]  DifferentiatorOutMax=[]  InitialConditionSetting=State (most efficient)
  cfblk9 : Delay
  cfblk2 : Outport
  cfblk8 : Outport  Port=2
  wires:
  cfblk6/1 -> cfblk2/1
  cfblk7/1 -> cfblk4/1
  cfblk1/1 -> cfblk6/1
  cfblk3/1 -> cfblk5/1
  cfblk4/1 -> cfblk8/1
  cfblk5/1 -> cfblk9/1
  cfblk9/1 -> cfblk3/1

== system sampleModel2432/cfblk241 ==
  cfblk1 : Inport
  cfblk8 : Inport  Port=2
  cfblk9 : Inport  Port=3
  cfblk10 : Inport  Port=4
  cfblk11 : Inport  Port=5
  Action Port : ActionPort  ActionType=then
  cfblk13 : Delay
  cfblk3 : Delay
  cfblk4 : Delay  ShowEnablePort=on
      settings: InputPortMap=u0,e6
  cfblk5 : UnitDelay  SampleTime=-1
  cfblk6 : Delay  ShowEnablePort=on
      settings: InputPortMap=u0,e6
  cfblk7 : DiscreteStateSpace  SampleTime=-1
  cfblk2 : Outport
  cfblk12 : Outport  Port=2
  wires:
  cfblk10/1 -> cfblk3/1
  cfblk5/1 -> cfblk7/1
  cfblk6/1 -> cfblk4/1
  cfblk9/1 -> cfblk2/1
  cfblk3/1 -> cfblk12/1
  cfblk8/1 -> cfblk5/1
  cfblk7/1 -> cfblk4/2
  cfblk1/1 -> cfblk6/2
  cfblk4/1 -> cfblk13/1
  cfblk13/1 -> cfblk6/1

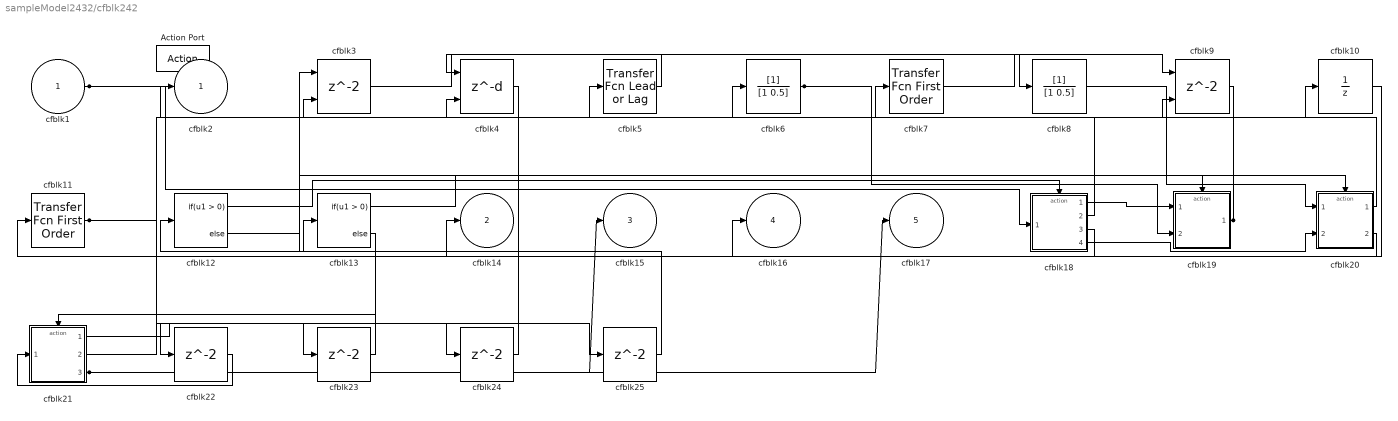
== system sampleModel2432/cfblk242 ==
  cfblk1 : Inport
  Action Port : ActionPort  ActionType=else
  cfblk10 : UnitDelay  SampleTime=-1
  cfblk11 : simulink/Discrete/Transfer Fcn First Order  PoleZ=0.95  ICPrevOutput=0.0  DoSatur=off
      settings: SourceProductName=Simulink
  cfblk12 : If  SampleTime=1
  cfblk13 : If  SampleTime=1
  cfblk18 : Subsystem  TreatAsAtomicUnit=on
  cfblk19 : Subsystem  TreatAsAtomicUnit=on
  cfblk20 : Subsystem  TreatAsAtomicUnit=on
  cfblk21 : Subsystem  TreatAsAtomicUnit=on
  cfblk{22..25} (4 alike) : Delay
  cfblk3 : Delay  ShowEnablePort=on
      settings: InputPortMap=u0,e6
  cfblk4 : Delay  DelayLengthSource=Input port
      settings: InputPortMap=u0,p1
  cfblk5 : simulink/Discrete/Transfer Fcn Lead or Lag  PoleZ=0.95  ZeroZ=0.75  ICPrevOutput=0.0  ICPrevInput=0.0  DoSatur=off
      settings: SourceProductName=Simulink  SourceProductBaseCode=SL
  cfblk6 : DiscreteFilter
  cfblk7 : simulink/Discrete/Transfer Fcn First Order  PoleZ=0.95  ICPrevOutput=0.0  DoSatur=off
      settings: SourceProductName=Simulink
  cfblk8 : DiscreteFilter
  cfblk9 : Delay  ShowEnablePort=on
      settings: InputPortMap=u0,e6
  cfblk2 : Outport
  cfblk14 : Outport  Port=2
  cfblk15 : Outport  Port=3
  cfblk16 : Outport  Port=4
  cfblk17 : Outport  Port=5
  wires:
  cfblk18/1(cfblk2) -> cfblk19/1(cfblk1)
  cfblk1/1 -> cfblk18/1(cfblk1), cfblk6/1
  cfblk20/1(cfblk2) -> cfblk5/1
  cfblk3/1 -> cfblk8/1
  cfblk10/1 -> cfblk16/1
  cfblk19/1(cfblk2) -> cfblk3/2, cfblk2/1
  cfblk5/1 -> cfblk4/1
  cfblk18/2(cfblk9) -> cfblk7/1
  cfblk6/1 -> cfblk19/2(cfblk10), cfblk9/2
  cfblk20/2(cfblk14) -> cfblk11/1
  cfblk8/1 -> cfblk20/1(cfblk1)
  cfblk9/1 -> cfblk4/2
  cfblk18/3(cfblk10) -> cfblk14/1
  cfblk11/1 -> cfblk10/1, cfblk25/1
  cfblk7/1 -> cfblk9/1
  cfblk21/3(cfblk16) -> cfblk15/1, cfblk17/1
  cfblk18/4(cfblk11) -> cfblk20/2(cfblk13)
  cfblk12/1 -> cfblk18/Action
  cfblk12/2 -> cfblk19/Action
  cfblk13/1 -> cfblk20/Action
  cfblk13/2 -> cfblk21/Action
  cfblk4/1 -> cfblk22/1
  cfblk22/1 -> cfblk21/1(cfblk1)
  cfblk21/1(cfblk2) -> cfblk23/1
  cfblk23/1 -> cfblk3/1
  cfblk21/2(cfblk15) -> cfblk24/1
  cfblk24/1 -> cfblk12/1
  cfblk25/1 -> cfblk13/1

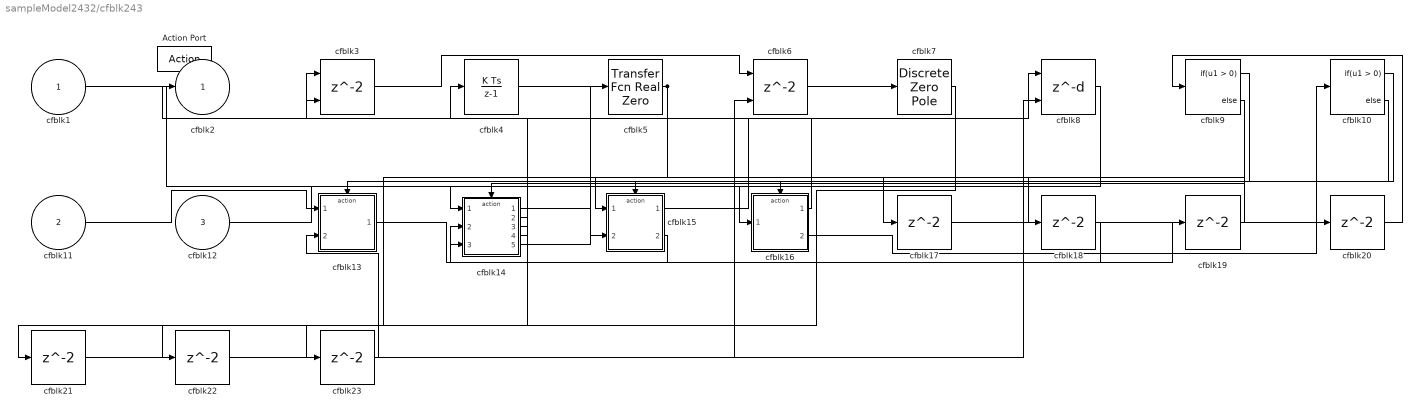
== system sampleModel2432/cfblk243 ==
  cfblk1 : Inport
  cfblk11 : Inport  Port=2
  cfblk12 : Inport  Port=3
  Action Port : ActionPort  ActionType=then
  cfblk10 : If  SampleTime=1
  cfblk13 : Subsystem  TreatAsAtomicUnit=on
  cfblk14 : Subsystem  TreatAsAtomicUnit=on
  cfblk15 : Subsystem  TreatAsAtomicUnit=on
  cfblk16 : Subsystem  TreatAsAtomicUnit=on
  cfblk{17..23} (7 alike) : Delay
  cfblk3 : Delay  ShowEnablePort=on
      settings: InputPortMap=u0,e6
  cfblk4 : DiscreteIntegrator  InitialConditionSetting=State (most efficient)  SampleTime=-1  ICPrevOutput=DiscIntNeverNeededParam  ICPrevScaledInput=DiscIntNeverNeededParam
  cfblk5 : simulink/Discrete/Transfer Fcn Real Zero  ZeroZ=0.75  ICPrevInput=0.0  DoSatur=off
      settings: SourceProductName=Simulink  SourceProductBaseCode=SL
  cfblk6 : Delay  ShowEnablePort=on
      settings: InputPortMap=u0,e6
  cfblk7 : DiscreteZeroPole  Poles=[0 0.5]  Gain=1  SampleTime=-1
  cfblk8 : Delay  DelayLengthSource=Input port
      settings: InputPortMap=u0,p1
  cfblk9 : If  SampleTime=1
  cfblk2 : Outport
  wires:
  cfblk16/1(cfblk2) -> cfblk4/1
  cfblk3/1 -> cfblk6/1
  cfblk12/1 -> cfblk16/1(cfblk1)
  cfblk11/1 -> cfblk13/1(cfblk1)
  cfblk5/1 -> cfblk2/1, cfblk23/1
  cfblk15/1(cfblk2) -> cfblk8/1
  cfblk8/1 -> cfblk14/1(cfblk1)
  cfblk6/1 -> cfblk7/1
  cfblk15/2(cfblk16) -> cfblk14/2(cfblk11)
  cfblk14/3(cfblk14) -> cfblk3/1
  cfblk14/4(cfblk15) -> cfblk3/2
  cfblk1/1 -> cfblk15/2(cfblk15)
  cfblk14/5(cfblk16) -> cfblk5/1
  cfblk9/1 -> cfblk13/Action
  cfblk9/2 -> cfblk14/Action
  cfblk10/1 -> cfblk15/Action
  cfblk10/2 -> cfblk16/Action
  cfblk14/1(cfblk2) -> cfblk17/1
  cfblk17/1 -> cfblk10/1
  cfblk4/1 -> cfblk18/1
  cfblk18/1 -> cfblk14/3(cfblk12)
  cfblk13/1(cfblk2) -> cfblk19/1
  cfblk19/1 -> cfblk15/1(cfblk1)
  cfblk16/2(cfblk14) -> cfblk20/1
  cfblk20/1 -> cfblk9/1
  cfblk14/2(cfblk13) -> cfblk21/1
  cfblk21/1 -> cfblk8/2
  cfblk7/1 -> cfblk22/1
  cfblk22/1 -> cfblk6/2
  cfblk23/1 -> cfblk13/2(cfblk10)

== system sampleModel2432/cfblk244 ==
  cfblk1 : Inport
  Action Port : ActionPort  ActionType=else
  cfblk10 : Subsystem  TreatAsAtomicUnit=on
  cfblk11 : Subsystem  TreatAsAtomicUnit=on
  cfblk{12..15} (4 alike) : Delay
  cfblk3 : simulink/Discrete/Transfer Fcn Lead or Lag  PoleZ=0.95  ZeroZ=0.75  ICPrevOutput=0.0  ICPrevInput=0.0  DoSatur=off
      settings: SourceProductName=Simulink  SourceProductBaseCode=SL
  cfblk4 : UnitDelay  SampleTime=-1
  cfblk5 : If  SampleTime=1
  cfblk6 : If  SampleTime=1
  cfblk8 : Subsystem  TreatAsAtomicUnit=on
  cfblk9 : Subsystem  TreatAsAtomicUnit=on
  cfblk2 : Outport
  cfblk7 : Outport  Port=2
  wires:
  cfblk3/1 -> cfblk9/3(cfblk9), cfblk12/1
  cfblk11/1(cfblk2) -> cfblk9/1(cfblk1)
  cfblk4/1 -> cfblk2/1, cfblk9/2(cfblk8), cfblk14/1, cfblk15/1
  cfblk10/1(cfblk2) -> cfblk3/1
  cfblk10/2(cfblk7) -> cfblk8/1(cfblk1), cfblk4/1, cfblk5/1, cfblk7/1
  cfblk1/1 -> cfblk6/1, cfblk10/1(cfblk1)
  cfblk9/1(cfblk2) -> cfblk8/2(cfblk7)
  cfblk5/1 -> cfblk8/Action
  cfblk5/2 -> cfblk9/Action
  cfblk6/1 -> cfblk10/Action
  cfblk6/2 -> cfblk11/Action
  cfblk12/1 -> cfblk11/2(cfblk10)
  cfblk8/1(cfblk2) -> cfblk13/1
  cfblk13/1 -> cfblk11/1(cfblk1)
  cfblk14/1 -> cfblk11/3(cfblk11)
  cfblk15/1 -> cfblk11/4(cfblk12)

== system sampleModel2432/cfblk196/cfblk12 ==
  cfblk1 : Inport
  cfblk10 : Inport  Port=2
  Action Port : ActionPort  ActionType=then
  cfblk3 : simulink/Discrete/Transfer Fcn First Order  PoleZ=0.95  ICPrevOutput=0.0  DoSatur=off
      settings: SourceProductName=Simulink
  cfblk4 : simulink/Discrete/Transfer Fcn First Order  PoleZ=0.95  ICPrevOutput=0.0  DoSatur=off
      settings: SourceProductName=Simulink
  cfblk5 : DiscreteFilter
  cfblk6 : Delay  ShowEnablePort=on
      settings: InputPortMap=u0,e6
  cfblk7 : simulink/Continuous/PID Controller (2DOF)  Controller=PID  TimeDomain=Discrete-time  SampleTime=-1  IntegratorMethod=Forward Euler  FilterMethod=Forward Euler  Form=Parallel  UseFilter=on  ControllerParametersSource=internal  P=1  I=1  D=0  N=100  b=1  c=1  InitialConditionSource=internal  InitialConditionForIntegrator=0  InitialConditionForFilter=0  ExternalReset=none  LimitOutput=off  UpperSaturationLimit=inf  LowerSaturationLimit=-inf  LinearizeAsGain=off  AntiWindupMode=none  Kb=1  TrackingMode=off  Kt=1  PParamMin=[]  PParamMax=[]  IParamMin=[]  IParamMax=[]  DParamMin=[]  DParamMax=[]  NParamMin=[]  NParamMax=[]  bParamMin=[]  bParamMax=[]  cParamMin=[]  cParamMax=[]  KbParamMin=[]  KbParamMax=[]  KtParamMin=[]  KtParamMax=[]  POutMin=[]  POutMax=[]  IOutMin=[]  IOutMax=[]  DOutMin=[]  DOutMax=[]  NOutMin=[]  NOutMax=[]  bOutMin=[]  bOutMax=[]  cOutMin=[]  cOutMax=[]  KbOutMin=[]  KbOutMax=[]  KtOutMin=[]  KtOutMax=[]  IntegratorOutMin=[]  IntegratorOutMax=[]  FilterOutMin=[]  FilterOutMax=[]  SumOutMin=[]  SumOutMax=[]  Sum1OutMin=[]  Sum1OutMax=[]  Sum2OutMin=[]  Sum2OutMax=[]  Sum3OutMin=[]  Sum3OutMax=[]  SumI1OutMin=[]  SumI1OutMax=[]  SumI2OutMin=[]  SumI2OutMax=[]  SumI3OutMin=[]  SumI3OutMax=[]  SumDOutMin=[]  SumDOutMax=[]  SaturationOutMin=[]  SaturationOutMax=[]  IntegratorContinuousStateAttributes=''  IntegratorStateMustResolveToSignalObject=off  IntegratorRTWStateStorageClass=Auto  FilterContinuousStateAttributes=''  FilterStateMustResolveToSignalObject=off  FilterRTWStateStorageClass=Auto  DifferentiatorICPrevScaledInput=0  DifferentiatorOutMin=[]  DifferentiatorOutMax=[]  InitialConditionSetting=State (most efficient)
  cfblk8 : UnitDelay  SampleTime=-1
  cfblk9 : UnitDelay  SampleTime=-1
  cfblk2 : Outport
  cfblk11 : Outport  Port=2
  cfblk12 : Outport  Port=3
  wires:
  cfblk3/1 -> cfblk5/1
  cfblk5/1 -> cfblk4/1, cfblk7/2
  cfblk1/1 -> cfblk8/1
  cfblk10/1 -> cfblk11/1
  cfblk9/1 -> cfblk3/1
  cfblk4/1 -> cfblk2/1
  cfblk8/1 -> cfblk6/1, cfblk7/1, cfblk9/1
  cfblk7/1 -> cfblk6/2
  cfblk6/1 -> cfblk12/1

== system sampleModel2432/cfblk196/cfblk13 ==
  cfblk1 : Inport
  cfblk8 : Inport  Port=2
  Action Port : ActionPort  ActionType=else
  cfblk3 : simulink/Discrete/Transfer Fcn Lead or Lag  PoleZ=0.95  ZeroZ=0.75  ICPrevOutput=0.0  ICPrevInput=0.0  DoSatur=off
      settings: SourceProductName=Simulink  SourceProductBaseCode=SL
  cfblk4 : UnitDelay  SampleTime=-1
  cfblk5 : Delay  DelayLengthSource=Input port
      settings: InputPortMap=u0,p1
  cfblk6 : DiscreteFir
  cfblk7 : simulink/Discrete/Tapped Delay  vinit=0.0  samptime=-1  NumDelays=1  DelayOrder=Oldest  includeCurrent=off
  cfblk2 : Outport
  cfblk9 : Outport  Port=2
  wires:
  cfblk1/1 -> cfblk4/1
  cfblk8/1 -> cfblk5/1
  cfblk4/1 -> cfblk7/1, cfblk6/1
  cfblk6/1 -> cfblk3/1
  cfblk3/1 -> cfblk9/1
  cfblk5/1 -> cfblk2/1
  cfblk7/1 -> cfblk5/2

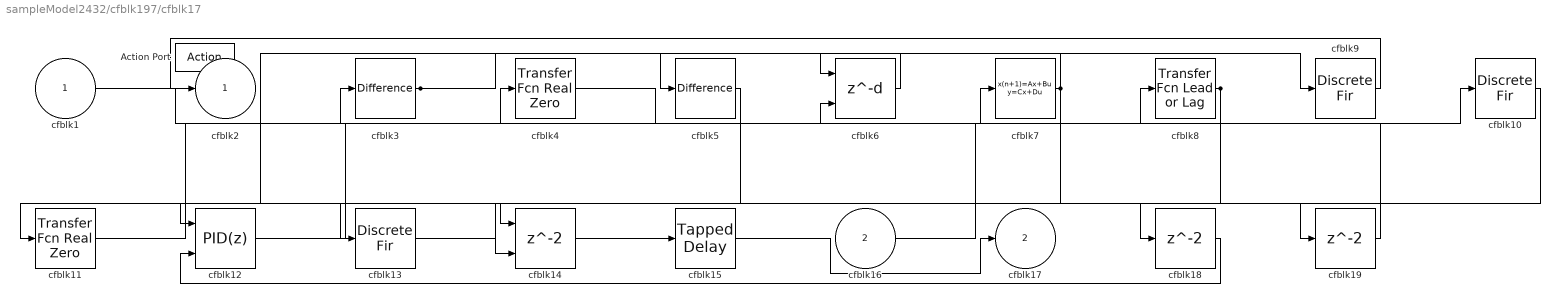
== system sampleModel2432/cfblk197/cfblk17 ==
  cfblk1 : Inport
  cfblk16 : Inport  Port=2
  Action Port : ActionPort  ActionType=then
  cfblk10 : DiscreteFir
  cfblk11 : simulink/Discrete/Transfer Fcn Real Zero  ZeroZ=0.75  ICPrevInput=0.0  DoSatur=off
      settings: SourceProductName=Simulink  SourceProductBaseCode=SL
  cfblk12 : simulink/Continuous/PID Controller (2DOF)  Controller=PID  TimeDomain=Discrete-time  SampleTime=-1  IntegratorMethod=Forward Euler  FilterMethod=Forward Euler  Form=Parallel  UseFilter=on  ControllerParametersSource=internal  P=1  I=1  D=0  N=100  b=1  c=1  InitialConditionSource=internal  InitialConditionForIntegrator=0  InitialConditionForFilter=0  ExternalReset=none  LimitOutput=off  UpperSaturationLimit=inf  LowerSaturationLimit=-inf  LinearizeAsGain=off  AntiWindupMode=none  Kb=1  TrackingMode=off  Kt=1  PParamMin=[]  PParamMax=[]  IParamMin=[]  IParamMax=[]  DParamMin=[]  DParamMax=[]  NParamMin=[]  NParamMax=[]  bParamMin=[]  bParamMax=[]  cParamMin=[]  cParamMax=[]  KbParamMin=[]  KbParamMax=[]  KtParamMin=[]  KtParamMax=[]  POutMin=[]  POutMax=[]  IOutMin=[]  IOutMax=[]  DOutMin=[]  DOutMax=[]  NOutMin=[]  NOutMax=[]  bOutMin=[]  bOutMax=[]  cOutMin=[]  cOutMax=[]  KbOutMin=[]  KbOutMax=[]  KtOutMin=[]  KtOutMax=[]  IntegratorOutMin=[]  IntegratorOutMax=[]  FilterOutMin=[]  FilterOutMax=[]  SumOutMin=[]  SumOutMax=[]  Sum1OutMin=[]  Sum1OutMax=[]  Sum2OutMin=[]  Sum2OutMax=[]  Sum3OutMin=[]  Sum3OutMax=[]  SumI1OutMin=[]  SumI1OutMax=[]  SumI2OutMin=[]  SumI2OutMax=[]  SumI3OutMin=[]  SumI3OutMax=[]  SumDOutMin=[]  SumDOutMax=[]  SaturationOutMin=[]  SaturationOutMax=[]  IntegratorContinuousStateAttributes=''  IntegratorStateMustResolveToSignalObject=off  IntegratorRTWStateStorageClass=Auto  FilterContinuousStateAttributes=''  FilterStateMustResolveToSignalObject=off  FilterRTWStateStorageClass=Auto  DifferentiatorICPrevScaledInput=0  DifferentiatorOutMin=[]  DifferentiatorOutMax=[]  InitialConditionSetting=State (most efficient)
  cfblk13 : DiscreteFir
  cfblk14 : Delay  ShowEnablePort=on
      settings: InputPortMap=u0,e6
  cfblk15 : simulink/Discrete/Tapped Delay  vinit=0.0  samptime=-1  NumDelays=1  DelayOrder=Oldest  includeCurrent=off
  cfblk18 : Delay
  cfblk19 : Delay
  cfblk3 : simulink/Discrete/Difference  ICPrevInput=0.0  OutMin=[]  OutMax=[]  OutDataTypeStr=Inherit: Inherit via back propagation  OutDataType=fixdt(1, 16)  OutScaling=2^-10  DoSatur=off
  cfblk4 : simulink/Discrete/Transfer Fcn Real Zero  ZeroZ=0.75  ICPrevInput=0.0  DoSatur=off
      settings: SourceProductName=Simulink  SourceProductBaseCode=SL
  cfblk5 : simulink/Discrete/Difference  ICPrevInput=0.0  OutMin=[]  OutMax=[]  OutDataTypeStr=Inherit: Inherit via back propagation  OutDataType=fixdt(1, 16)  OutScaling=2^-10  DoSatur=off
  cfblk6 : Delay  DelayLengthSource=Input port
      settings: InputPortMap=u0,p1
  cfblk7 : DiscreteStateSpace  SampleTime=-1
  cfblk8 : simulink/Discrete/Transfer Fcn Lead or Lag  PoleZ=0.95  ZeroZ=0.75  ICPrevOutput=0.0  ICPrevInput=0.0  DoSatur=off
      settings: SourceProductName=Simulink  SourceProductBaseCode=SL
  cfblk9 : DiscreteFir
  cfblk2 : Outport
  cfblk17 : Outport  Port=2
  wires:
  cfblk14/1 -> cfblk15/1
  cfblk10/1 -> cfblk14/1
  cfblk12/1 -> cfblk8/1
  cfblk15/1 -> cfblk17/1
  cfblk7/1 -> cfblk11/1, cfblk13/1
  cfblk6/1 -> cfblk5/1
  cfblk9/1 -> cfblk2/1
  cfblk11/1 -> cfblk3/1
  cfblk1/1 -> cfblk4/1
  cfblk3/1 -> cfblk6/1, cfblk9/1
  cfblk5/1 -> cfblk12/1
  cfblk16/1 -> cfblk10/1
  cfblk8/1 -> cfblk14/2, cfblk18/1
  cfblk4/1 -> cfblk6/2
  cfblk18/1 -> cfblk12/2
  cfblk13/1 -> cfblk19/1
  cfblk19/1 -> cfblk7/1
